simulink model "MRAC_proyecto_Arduino"  (R2024b)
settings: Solver=FixedStepDiscrete  StartTime=0.0  StopTime=inf  FixedStep=Ts_MRAC_Arduino  RelTol=1e-6  EnableMultiTasking=on
undefined symbols (not defined in the file or in its folder): adapt_enable_MRAC, Amd_MRAC, Bmd_MRAC, control_enable_MRAC, deg2rad_MRAC, DiscIntNeverNeededParam, Gamma_r_MRAC, Gamma_x_MRAC, gyro_bias_dps_MRAC, gyro_sign_MRAC, Kr0_Arduino_MRAC, KxT0_Arduino_MRAC, PB_MRAC, Ts_MRAC_Arduino, u_max_MRAC, u_min_MRAC
libraries: arduinolib x2, arduinosensorlib x1
settings Model: SimulationMode=external  ExtModeTrigDuration=2  Creator=juanm  LastModifiedBy=juanm
settings SolverCC: AutoInsertRateTranBlk=on
settings OptimizationCC: EnhancedBackFolding=on  PassReuseOutputArgsAs=Individual arguments  ZeroExternalMemoryAtStartup=off  ZeroInternalMemoryAtStartup=off  MaxStackSize=64  OptimizeBlockOrder=speed  DifferentSizesBufferReuse=on  OptimizationCustomize=off  EfficientTunableParamExpr=on
settings DebuggingCC: ParameterTunabilityLossMsg=error
settings HardwareCC: ProdBitPerInt=16  ProdBitPerPointer=16  ProdBitPerSizeT=16  ProdBitPerPtrDiffT=16  ProdLargestAtomicFloat=None  ProdWordSize=8  ProdHWDeviceType=Atmel->AVR  UseEmbeddedCoderFeatures=off  UseSimulinkCoderFeatures=off
settings SFSimCC: MATLABDynamicMemAlloc=off
settings RTWCC: Description=Embedded Coder  SystemTargetFile=ert.tlc  HardwareBoard=Arduino Uno  TemplateMakefile=ert_default_tmf  Toolchain=Arduino AVR  BuildConfiguration=Faster Runs
settings CodeAppCC: ForceParamTrailComments=on  IgnoreCustomStorageClasses=off  OperatorAnnotations=on  SimulinkDataObjDesc=on  SFDataObjDesc=on  InsertBlockDesc=on
settings ERTTargetCC: SupportContinuousTime=on  SupportNonInlinedSFcns=on  SupportVariableSizeSignals=on  ExtModeTransport=3  ExtModeStaticAlloc=on  ExtModeAutomaticAllocSize=off  ExtModeStaticAllocSize=250  ExtModeMexFile=ext_xcp  ExtModeIntrfLevel=Level2 - Open  InlinedParameterPlacement=Hierarchical

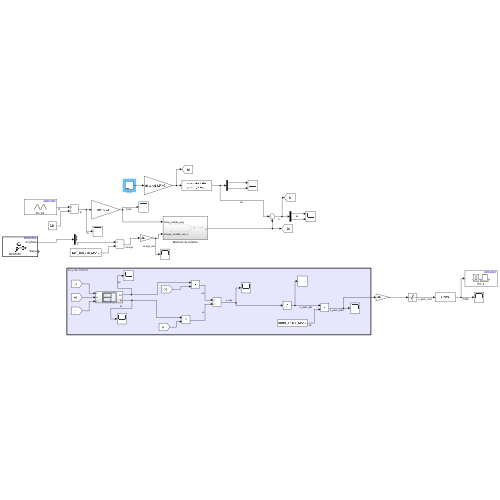
[thumbnail: Simulink's stored preview of the top-level diagram]
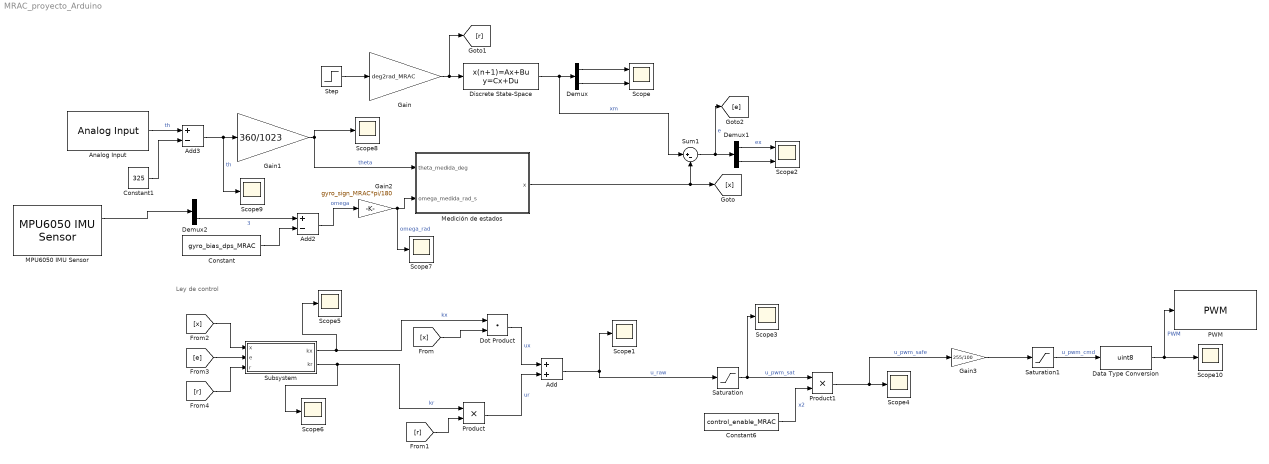
== system MRAC_proyecto_Arduino ==
  note: Ley de control
  Add : Sum
  Add2 : Sum  Inputs=+-
  Add3 : Sum  Inputs=+-
  Analog Input : arduinolib/Analog Input  pinNumber=3  ReadResultsOnly=off  ConversionTriggerSource=Software  ExternalTriggerType=uint32( 0 )  OutputDataType=uint16  EnableConversionCompleteNotify=off  EnableOuputStatus=off  SampleTime=-1  blockPlatform=arduino
      settings: SourceProductName=Common
  Constant : Constant  Value=gyro_bias_dps_MRAC
  Constant1 : Constant  Value=325
  Constant6 : Constant  Value=control_enable_MRAC
  Data Type Conversion : DataTypeConversion  OutDataTypeStr=uint8  SaturateOnIntegerOverflow=off  RndMeth=Floor
  Demux : Demux  Outputs=2
  Demux1 : Demux  Outputs=2
  Demux2 : Demux  Outputs=3
  Discrete State-Space : DiscreteStateSpace  A=Amd_MRAC  B=Bmd_MRAC  C=eye(2)  D=zeros(2,1)  InitialCondition=[0;0]  SampleTime=Ts_MRAC_Arduino
  Dot Product : DotProduct  OutDataTypeStr=Inherit: Inherit via internal rule
  Gain : Gain  Gain=deg2rad_MRAC
  Gain1 : Gain  Gain=360/1023
  Gain2 : Gain  Gain=gyro_sign_MRAC*pi/180
  Gain3 : Gain  Gain=255/100
  MPU6050 IMU Sensor : arduinosensorlib/MPU6050 IMU Sensor  I2CModule=0  SlaveAddress=0x68  Accel=off  AngularRate=on  Temperature=off  Status=on  Timestamp=off  EulerAngles=off  Quat=off  AccelRange=2G  GyroRange=250 dps  DmpOdr=200 Hz  Dlpf=Accelerometer: 184Hz, Gyroscope: 188Hz  spf=1  SampleTime=Ts_MRAC_Arduino  QueueSizeFactor=1
      settings: SourceProductName=Sensors
  Medición de estados : Subsystem
  PWM : arduinolib/PWM  pinNumber=9  frequencyType=Default  desiredFrequency=490.2  achievableFrequency=490.2
      settings: SourceProductName=Common
  Product : Product
  Product1 : Product
  Saturation : Saturate  UpperLimit=u_max_MRAC  LowerLimit=u_min_MRAC
  Saturation1 : Saturate  UpperLimit=255  LowerLimit=0
  Scope : Scope  NumInputPorts=2
  Scope{1,3..10} (9 alike) : Scope
  Scope2 : Scope  NumInputPorts=2
  Step : Step  After=110  SampleTime=Ts_MRAC_Arduino
  Subsystem : Subsystem
  Sum1 : Sum  Inputs=|+-
  wires:
  Step/1 -> Gain/1
  Discrete State-Space/1 -> Sum1/1, Demux/1  "xm"
  Gain/1 -> [r], Discrete State-Space/1
  Demux/1 -> Scope/1
  Demux/2 -> Scope/2
  Sum1/1 -> [e], Demux1/1  "e"
  Demux1/1 -> Scope2/1  "ex"
  Demux1/2 -> Scope2/2
  Subsystem/1(kx) -> Scope5/1, Dot Product/1  "kx"
  [x] -> Dot Product/2
  Subsystem/2(kr) -> Scope6/1, Product/1  "kr"
  [r] -> Product/2
  Dot Product/1 -> Add/1  "ux"
  Product/1 -> Add/2  "ur"
  Add/1 -> Saturation/1, Scope1/1  "u_raw"
  Saturation/1 -> Scope3/1, Product1/1  "u_pwm_sat"
  Constant6/1 -> Product1/2  "x2"
  Product1/1 -> Gain3/1, Scope4/1  "u_pwm_safe"
  [x] -> Subsystem/1(x)
  [e] -> Subsystem/2(e)
  [r] -> Subsystem/3(r)
  Demux2/3 -> Add2/1  "3"
  Medición de estados/1(x) -> Sum1/2, [x]
  Gain1/1 -> Scope8/1, Medición de estados/1(theta_medida_deg)  "theta"
  Analog Input/1 -> Add3/1  "th"
  MPU6050 IMU Sensor/1 -> Demux2/1
  Constant/1 -> Add2/2
  Add2/1 -> Gain2/1  "omega"
  Gain2/1 -> Scope7/1, Medición de estados/2(omega_medida_rad_s)  "omega_rad"
  Constant1/1 -> Add3/2
  Add3/1 -> Scope9/1, Gain1/1  "th"
  Gain3/1 -> Saturation1/1
  Saturation1/1 -> Data Type Conversion/1  "u_pwm_cmd"
  Data Type Conversion/1 -> PWM/1, Scope10/1  "PWM"

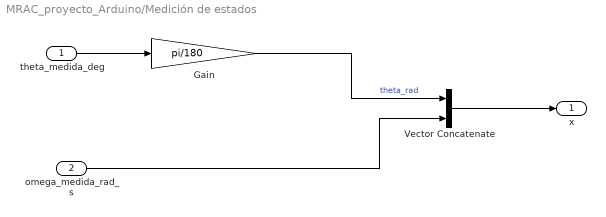
== system MRAC_proyecto_Arduino/Medición de estados ==
  theta_medida_deg : Inport
  omega_medida_rad_s : Inport  Port=2
  Gain : Gain  Gain=pi/180
  Vector Concatenate : Concatenate
  x : Outport
  wires:
  theta_medida_deg/1 -> Gain/1
  Gain/1 -> Vector Concatenate/1  "theta_rad"
  omega_medida_rad_s/1 -> Vector Concatenate/2
  Vector Concatenate/1 -> x/1

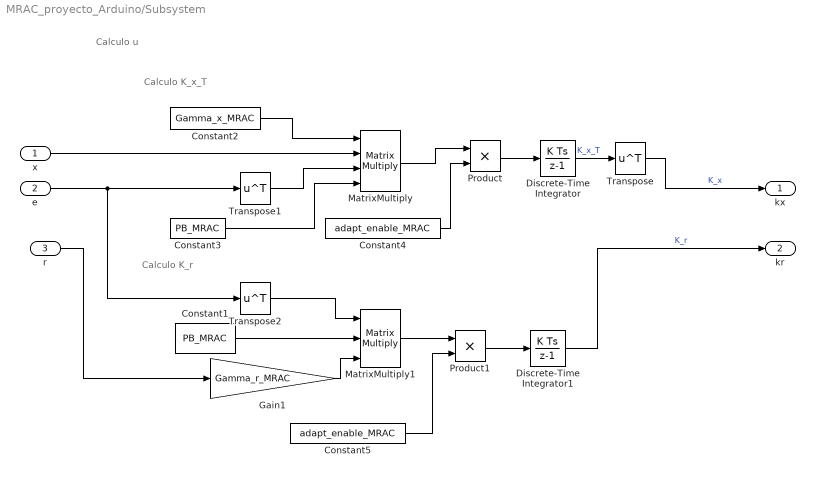
== system MRAC_proyecto_Arduino/Subsystem ==
  note: Calculo K_r
  note: Calculo K_x_T
  note: Calculo u
  x : Inport
  e : Inport  Port=2
  r : Inport  Port=3
  Constant1 : Constant  Value=PB_MRAC
  Constant2 : Constant  Value=Gamma_x_MRAC
  Constant3 : Constant  Value=PB_MRAC
  Constant4 : Constant  Value=adapt_enable_MRAC
  Constant5 : Constant  Value=adapt_enable_MRAC
  Discrete-Time Integrator : DiscreteIntegrator  InitialCondition=KxT0_Arduino_MRAC  SampleTime=Ts_MRAC_Arduino  ICPrevOutput=DiscIntNeverNeededParam  ICPrevScaledInput=DiscIntNeverNeededParam
  Discrete-Time Integrator1 : DiscreteIntegrator  InitialCondition=Kr0_Arduino_MRAC  SampleTime=Ts_MRAC_Arduino  ICPrevOutput=DiscIntNeverNeededParam  ICPrevScaledInput=DiscIntNeverNeededParam
  Gain1 : Gain  Gain=Gamma_r_MRAC
  MatrixMultiply : Product  Inputs=4  Multiplication=Matrix(*)
  MatrixMultiply1 : Product  Inputs=3  Multiplication=Matrix(*)
  Product : Product
  Product1 : Product
  Transpose : Math  Operator=transpose
  Transpose1 : Math  Operator=transpose
  Transpose2 : Math  Operator=transpose
  kx : Outport
  kr : Outport  Port=2
  wires:
  Discrete-Time Integrator1/1 -> kr/1  "K_r"
  Discrete-Time Integrator/1 -> Transpose/1  "K_x_T"
  MatrixMultiply/1 -> Product/1
  Transpose/1 -> kx/1  "K_x"
  Gain1/1 -> MatrixMultiply1/3
  Constant3/1 -> MatrixMultiply/4
  Transpose2/1 -> MatrixMultiply1/1
  MatrixMultiply1/1 -> Product1/1
  Constant1/1 -> MatrixMultiply1/2
  Constant2/1 -> MatrixMultiply/1
  r/1 -> Gain1/1
  e/1 -> Transpose2/1, Transpose1/1
  x/1 -> MatrixMultiply/2
  Transpose1/1 -> MatrixMultiply/3
  Product/1 -> Discrete-Time Integrator/1
  Constant4/1 -> Product/2
  Constant5/1 -> Product1/2
  Product1/1 -> Discrete-Time Integrator1/1
